simulink model "store"  (R2017b)
settings: Solver=VariableStepAuto  StartTime=0.0  StopTime=10.0  RelTol=1e-3
libraries: simulink x1
settings Model: Creator=Administrator  LastModifiedBy=Administrator

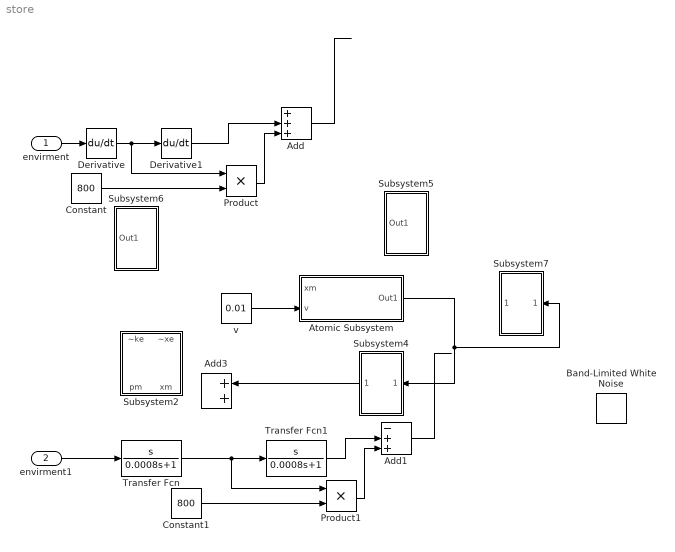
== system store ==
  envirment : Inport
  envirment1 : Inport  Port=2
  Add : Sum  Inputs=+++
  Add1 : Sum  Inputs=-++
  Add3 : Sum
  Atomic Subsystem : Subsystem  TreatAsAtomicUnit=on
  Band-Limited White Noise : simulink/Sources/Band-Limited White Noise  Cov=[0.000000005]  Ts=0.005  seed=[23341]
  Constant : Constant  Value=800
  Constant1 : Constant  Value=800
  Derivative : Derivative
  Derivative1 : Derivative
  Product : Product
  Product1 : Product
  Subsystem2 : Subsystem
  Subsystem4 : Subsystem
  Subsystem5 : Subsystem
  Subsystem6 : Subsystem
  Subsystem7 : Subsystem
  Transfer Fcn : TransferFcn  Numerator=[1 0]  Denominator=[0.0008 1]
  Transfer Fcn1 : TransferFcn  Numerator=[1 0]  Denominator=[0.0008 1]
  v : Constant  Value=0.01
  wires:
  v/1 -> Atomic Subsystem/2(v)
  Atomic Subsystem/1(Out1) -> Subsystem7/1(In1), Subsystem4/1(In1)
  Subsystem4/1(Out1) -> Add3/1
  envirment/1 -> Derivative/1
  ? -> Add/1
  Constant/1 -> Product/2
  Derivative/1 -> Product/1, Derivative1/1
  Add/1 -> ?
  Derivative1/1 -> Add/2
  Product/1 -> Add/3
  ? -> Add1/1
  envirment1/1 -> Transfer Fcn/1
  Transfer Fcn1/1 -> Add1/2
  Transfer Fcn/1 -> Transfer Fcn1/1, Product1/1
  Product1/1 -> Add1/3
  Add1/1 -> ?
  Constant1/1 -> Product1/2

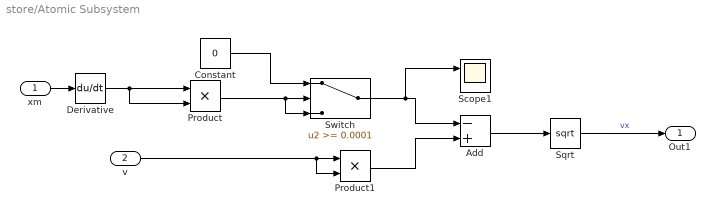
== system store/Atomic Subsystem ==
  xm : Inport
  v : Inport  Port=2
  Add : Sum  Inputs=-+
  Constant : Constant  Value=0
  Derivative : Derivative
  Product : Product
  Product1 : Product
  Scope1 : Scope  NumInputPorts=2
  Sqrt : Sqrt  SaturateOnIntegerOverflow=on
  Switch : Switch  Threshold=0.0001
  Out1 : Outport
  wires:
  xm/1 -> Derivative/1
  v/1 -> Product1/2, Product1/1
  Product1/1 -> Add/2
  Add/1 -> Sqrt/1
  Sqrt/1 -> Out1/1  "vx"
  Derivative/1 -> Product/2, Product/1
  Switch/1 -> Scope1/1, Add/1
  Constant/1 -> Switch/1
  Product/1 -> Switch/3, Switch/2

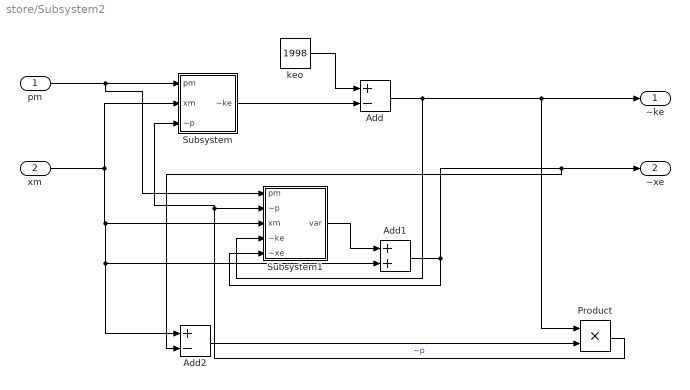
== system store/Subsystem2 ==
  pm : Inport
  xm : Inport  Port=2
  Add : Sum  Inputs=+-
  Add1 : Sum
  Add2 : Sum  Inputs=+-
  Product : Product
  Subsystem : Subsystem
  Subsystem1 : Subsystem
  keo : Constant  Value=1998
  ~ke : Outport
  ~xe : Outport  Port=2
  wires:
  pm/1 -> Subsystem1/1(pm), Subsystem/1(pm)
  xm/1 -> Subsystem/2(xm), Add1/2, Add2/1, Subsystem1/3(xm)
  Add/1 -> Subsystem1/4(~ke), Product/1, ~ke/1
  Subsystem/1(~ke) -> Add/2
  Subsystem1/1(var) -> Add1/1
  Add1/1 -> Subsystem1/5("~xe "), Add2/2, ~xe/1
  Add2/1 -> Product/2
  Product/1 -> Subsystem/3(~p), Subsystem1/2(~p)  "~p"
  keo/1 -> Add/1

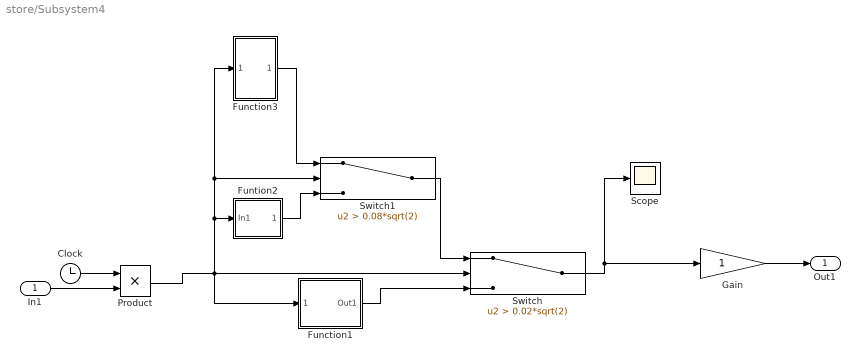
== system store/Subsystem4 ==
  In1 : Inport
  Clock : Clock
  Function1 : Subsystem
  Function3 : Subsystem
  Funtion2 : Subsystem
  Gain : Gain
  Product : Product
  Scope : Scope
  Switch : Switch  Criteria=u2 > Threshold  Threshold=0.02*sqrt(2)
  Switch1 : Switch  Criteria=u2 > Threshold  Threshold=0.08*sqrt(2)
  Out1 : Outport
  wires:
  Function3/1(Out1) -> Switch1/1
  Funtion2/1(Out1) -> Switch1/3
  Clock/1 -> Product/1
  Product/1 -> Function1/1(time in), Switch/2, Function3/1(In1), Switch1/2, Funtion2/1(In1)
  Switch1/1 -> Switch/1
  Switch/1 -> Gain/1, Scope/1
  Function1/1(Out1) -> Switch/3
  Gain/1 -> Out1/1
  In1/1 -> Product/2

== system store/Subsystem5 ==
  Clock : Clock
  Function1 : Subsystem
  Function3 : Subsystem
  Funtion2 : Subsystem
  Gain : Gain
  Gain1 : Gain  Gain=5/1000
  Scope : Scope
  Switch : Switch  Criteria=u2 > Threshold  Threshold=0.0282842712474619
  Switch1 : Switch  Criteria=u2 > Threshold  Threshold=0.1131370849898476
  Out1 : Outport
  wires:
  Gain/1 -> Out1/1
  Function1/1(Out1) -> Switch/3
  Switch/1 -> Scope/1, Gain/1
  Switch1/1 -> Switch/1
  Clock/1 -> Gain1/1
  Funtion2/1(Out1) -> Switch1/3
  Function3/1(Out1) -> Switch1/1
  Gain1/1 -> Funtion2/1(In1), Switch1/2, Function3/1(In1), Switch/2, Function1/1(time in)

== system store/Subsystem6 ==
  Clock : Clock
  Function1 : Subsystem
  Function3 : Subsystem
  Funtion2 : Subsystem
  Gain : Gain
  Gain1 : Gain  Gain=5/1000
  Scope : Scope
  Switch : Switch  Criteria=u2 > Threshold  Threshold=0.02*sqrt(2)
  Switch1 : Switch  Criteria=u2 > Threshold  Threshold=0.08*sqrt(2)
  Out1 : Outport
  wires:
  Gain/1 -> Out1/1
  Function1/1(Out1) -> Switch/3
  Switch/1 -> Scope/1, Gain/1
  Switch1/1 -> Switch/1
  Clock/1 -> Gain1/1
  Funtion2/1(Out1) -> Switch1/3
  Function3/1(Out1) -> Switch1/1
  Gain1/1 -> Funtion2/1(In1), Switch1/2, Function3/1(In1), Switch/2, Function1/1(time in)

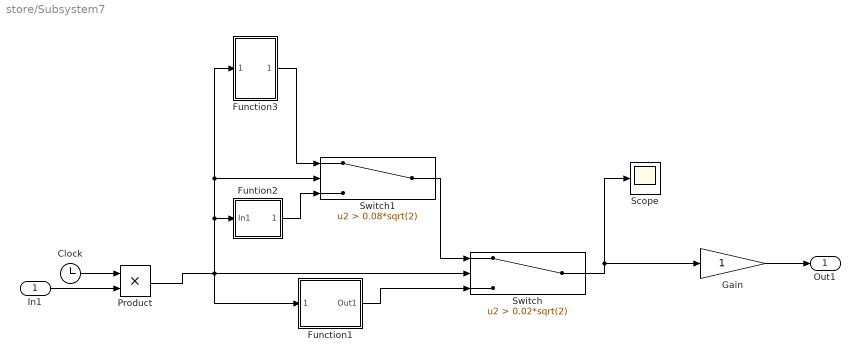
== system store/Subsystem7 ==
  In1 : Inport
  Clock : Clock
  Function1 : Subsystem
  Function3 : Subsystem
  Funtion2 : Subsystem
  Gain : Gain
  Product : Product
  Scope : Scope
  Switch : Switch  Criteria=u2 > Threshold  Threshold=0.02*sqrt(2)
  Switch1 : Switch  Criteria=u2 > Threshold  Threshold=0.08*sqrt(2)
  Out1 : Outport
  wires:
  In1/1 -> Product/2
  Gain/1 -> Out1/1
  Function1/1(Out1) -> Switch/3
  Switch/1 -> Scope/1, Gain/1
  Switch1/1 -> Switch/1
  Product/1 -> Funtion2/1(In1), Switch1/2, Function3/1(In1), Switch/2, Function1/1(time in)
  Clock/1 -> Product/1
  Funtion2/1(Out1) -> Switch1/3
  Function3/1(Out1) -> Switch1/1

== system store/Subsystem2/Subsystem ==
  pm : Inport
  xm : Inport  Port=2
  ~p : Inport  Port=3
  Add : Sum  Inputs=-+
  Integrator : Integrator
  Product : Product
  Product1 : Product
  Scope : Scope
  Subsystem1 : Subsystem
  ~ke : Outport
  wires:
  Subsystem1/2(γ2) -> Scope/1
  ~p/1 -> Add/2
  pm/1 -> Add/1
  xm/1 -> Product/1
  Add/1 -> Product/2
  Product/1 -> Integrator/1
  Integrator/1 -> Product1/2
  Product1/1 -> ~ke/1
  Subsystem1/1(γ1) -> Product1/1

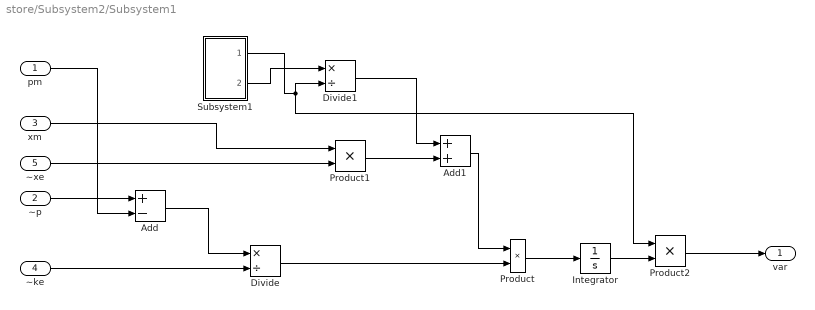
== system store/Subsystem2/Subsystem1 ==
  pm : Inport
  ~p : Inport  Port=2
  xm : Inport  Port=3
  ~ke : Inport  Port=4
  "~xe " : Inport  Port=5
  Add : Sum  Inputs=+-
  Add1 : Sum
  Divide : Product  Inputs=*/
  Divide1 : Product  Inputs=*/
  Integrator : Integrator
  Product : Product
  Product1 : Product
  Product2 : Product
  Subsystem1 : Subsystem
  var : Outport
  wires:
  pm/1 -> Add/2
  ~p/1 -> Add/1
  Add/1 -> Divide/1
  ~ke/1 -> Divide/2
  Divide/1 -> Product/2
  xm/1 -> Product1/1
  Divide1/1 -> Add1/1
  Product1/1 -> Add1/2
  Add1/1 -> Product/1
  Integrator/1 -> Product2/2
  Product2/1 -> var/1
  "~xe "/1 -> Product1/2
  Product/1 -> Integrator/1
  Subsystem1/2(gama2) -> Divide1/1
  Subsystem1/1(gama1) -> Product2/1, Divide1/2

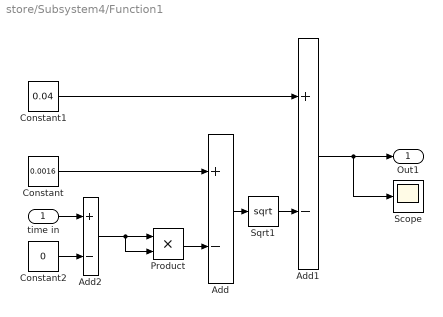
== system store/Subsystem4/Function1 ==
  time in : Inport
  Add : Sum  Inputs=+-
  Add1 : Sum  Inputs=+-
  Add2 : Sum  Inputs=+-
  Constant : Constant  Value=0.0016
  Constant1 : Constant  Value=0.04
  Constant2 : Constant  Value=0
  Product : Product
  Scope : Scope
  Sqrt1 : Sqrt  SaturateOnIntegerOverflow=on
  Out1 : Outport
  wires:
  Constant/1 -> Add/1
  time in/1 -> Add2/1
  Constant2/1 -> Add2/2
  Add2/1 -> Product/2, Product/1
  Product/1 -> Add/2
  Add/1 -> Sqrt1/1
  Sqrt1/1 -> Add1/2
  Constant1/1 -> Add1/1
  Add1/1 -> Out1/1, Scope/1

== system store/Subsystem4/Function3 ==
  In1 : Inport
  Add : Sum  Inputs=+-
  Add1 : Sum  Inputs=+-
  Add2 : Sum  Inputs=+-
  Product1 : Product
  Sqrt : Sqrt  SaturateOnIntegerOverflow=on
  pr2 : Constant  Value=0.0016
  pr3 : Constant  Value=0.1*sqrt(2)
  pr4 : Constant  Value=0.04
  Out1 : Outport
  wires:
  Add2/1 -> Out1/1
  pr3/1 -> Add1/2
  In1/1 -> Add1/1
  Add1/1 -> Product1/2, Product1/1
  Product1/1 -> Add/2
  pr2/1 -> Add/1
  Add/1 -> Sqrt/1
  pr4/1 -> Add2/1
  Sqrt/1 -> Add2/2

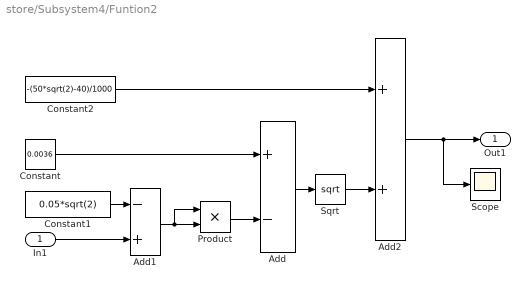
== system store/Subsystem4/Funtion2 ==
  In1 : Inport
  Add : Sum  Inputs=+-
  Add1 : Sum  Inputs=-+
  Add2 : Sum
  Constant : Constant  Value=0.0036
  Constant1 : Constant  Value=0.05*sqrt(2)
  Constant2 : Constant  Value=-(50*sqrt(2)-40)/1000
  Product : Product
  Scope : Scope
  Sqrt : Sqrt  SaturateOnIntegerOverflow=on
  Out1 : Outport
  wires:
  Constant/1 -> Add/1
  In1/1 -> Add1/2
  Add1/1 -> Product/1, Product/2
  Product/1 -> Add/2
  Constant1/1 -> Add1/1
  Add/1 -> Sqrt/1
  Sqrt/1 -> Add2/2
  Constant2/1 -> Add2/1
  Add2/1 -> Scope/1, Out1/1

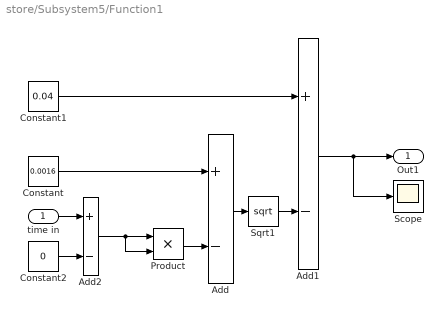
== system store/Subsystem5/Function1 ==
  time in : Inport
  Add : Sum  Inputs=+-
  Add1 : Sum  Inputs=+-
  Add2 : Sum  Inputs=+-
  Constant : Constant  Value=0.0016
  Constant1 : Constant  Value=0.04
  Constant2 : Constant  Value=0
  Product : Product
  Scope : Scope
  Sqrt1 : Sqrt  SaturateOnIntegerOverflow=on
  Out1 : Outport
  wires:
  Add1/1 -> Scope/1, Out1/1
  Constant1/1 -> Add1/1
  Sqrt1/1 -> Add1/2
  Add/1 -> Sqrt1/1
  Product/1 -> Add/2
  Add2/1 -> Product/1, Product/2
  Constant2/1 -> Add2/2
  time in/1 -> Add2/1
  Constant/1 -> Add/1

== system store/Subsystem5/Function3 ==
  In1 : Inport
  Add : Sum  Inputs=+-
  Add1 : Sum  Inputs=+-
  Add2 : Sum  Inputs=+-
  Product1 : Product
  Sqrt : Sqrt  SaturateOnIntegerOverflow=on
  pr2 : Constant  Value=0.0016
  pr3 : Constant  Value=0.14142135623731
  pr4 : Constant  Value=0.04
  Out1 : Outport
  wires:
  Sqrt/1 -> Add2/2
  pr4/1 -> Add2/1
  Add/1 -> Sqrt/1
  pr2/1 -> Add/1
  Product1/1 -> Add/2
  Add1/1 -> Product1/1, Product1/2
  In1/1 -> Add1/1
  pr3/1 -> Add1/2
  Add2/1 -> Out1/1

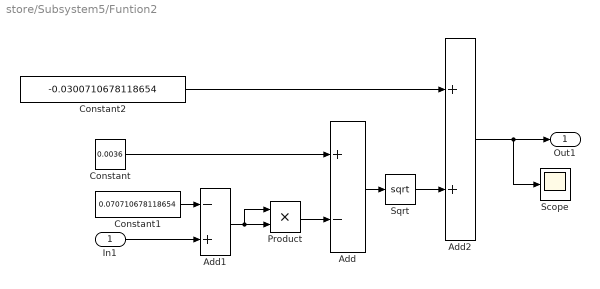
== system store/Subsystem5/Funtion2 ==
  In1 : Inport
  Add : Sum  Inputs=+-
  Add1 : Sum  Inputs=-+
  Add2 : Sum
  Constant : Constant  Value=0.0036
  Constant1 : Constant  Value=0.070710678118654
  Constant2 : Constant  Value=-0.0300710678118654
  Product : Product
  Scope : Scope
  Sqrt : Sqrt  SaturateOnIntegerOverflow=on
  Out1 : Outport
  wires:
  Add2/1 -> Out1/1, Scope/1
  Constant2/1 -> Add2/1
  Sqrt/1 -> Add2/2
  Add/1 -> Sqrt/1
  Constant1/1 -> Add1/1
  Product/1 -> Add/2
  Add1/1 -> Product/2, Product/1
  In1/1 -> Add1/2
  Constant/1 -> Add/1

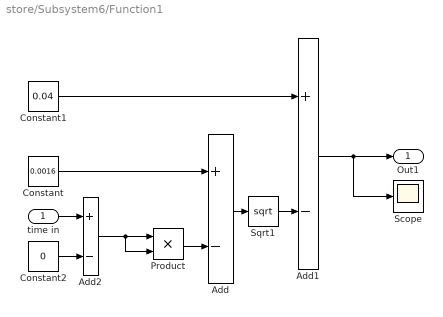
== system store/Subsystem6/Function1 ==
  time in : Inport
  Add : Sum  Inputs=+-
  Add1 : Sum  Inputs=+-
  Add2 : Sum  Inputs=+-
  Constant : Constant  Value=0.0016
  Constant1 : Constant  Value=0.04
  Constant2 : Constant  Value=0
  Product : Product
  Scope : Scope
  Sqrt1 : Sqrt  SaturateOnIntegerOverflow=on
  Out1 : Outport
  wires:
  Add1/1 -> Scope/1, Out1/1
  Constant1/1 -> Add1/1
  Sqrt1/1 -> Add1/2
  Add/1 -> Sqrt1/1
  Product/1 -> Add/2
  Add2/1 -> Product/1, Product/2
  Constant2/1 -> Add2/2
  time in/1 -> Add2/1
  Constant/1 -> Add/1

== system store/Subsystem6/Function3 ==
  In1 : Inport
  Add : Sum  Inputs=+-
  Add1 : Sum  Inputs=+-
  Add2 : Sum  Inputs=+-
  Product1 : Product
  Sqrt : Sqrt  SaturateOnIntegerOverflow=on
  pr2 : Constant  Value=0.0016
  pr3 : Constant  Value=0.1*sqrt(2)
  pr4 : Constant  Value=0.04
  Out1 : Outport
  wires:
  Sqrt/1 -> Add2/2
  pr4/1 -> Add2/1
  Add/1 -> Sqrt/1
  pr2/1 -> Add/1
  Product1/1 -> Add/2
  Add1/1 -> Product1/1, Product1/2
  In1/1 -> Add1/1
  pr3/1 -> Add1/2
  Add2/1 -> Out1/1

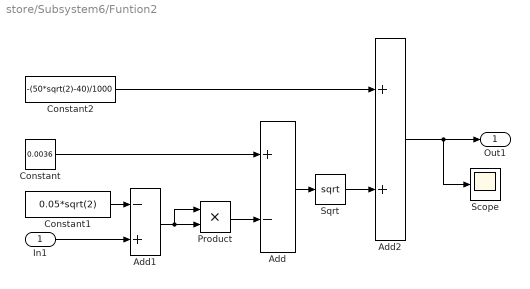
== system store/Subsystem6/Funtion2 ==
  In1 : Inport
  Add : Sum  Inputs=+-
  Add1 : Sum  Inputs=-+
  Add2 : Sum
  Constant : Constant  Value=0.0036
  Constant1 : Constant  Value=0.05*sqrt(2)
  Constant2 : Constant  Value=-(50*sqrt(2)-40)/1000
  Product : Product
  Scope : Scope
  Sqrt : Sqrt  SaturateOnIntegerOverflow=on
  Out1 : Outport
  wires:
  Add2/1 -> Out1/1, Scope/1
  Constant2/1 -> Add2/1
  Sqrt/1 -> Add2/2
  Add/1 -> Sqrt/1
  Constant1/1 -> Add1/1
  Product/1 -> Add/2
  Add1/1 -> Product/2, Product/1
  In1/1 -> Add1/2
  Constant/1 -> Add/1

== system store/Subsystem7/Function1 ==
  time in : Inport
  Add : Sum  Inputs=+-
  Add1 : Sum  Inputs=+-
  Add2 : Sum  Inputs=+-
  Constant : Constant  Value=0.0016
  Constant1 : Constant  Value=0.04
  Constant2 : Constant  Value=0
  Product : Product
  Scope : Scope
  Sqrt1 : Sqrt  SaturateOnIntegerOverflow=on
  Out1 : Outport
  wires:
  Add1/1 -> Scope/1, Out1/1
  Constant1/1 -> Add1/1
  Sqrt1/1 -> Add1/2
  Add/1 -> Sqrt1/1
  Product/1 -> Add/2
  Add2/1 -> Product/1, Product/2
  Constant2/1 -> Add2/2
  time in/1 -> Add2/1
  Constant/1 -> Add/1

== system store/Subsystem7/Function3 ==
  In1 : Inport
  Add : Sum  Inputs=+-
  Add1 : Sum  Inputs=+-
  Add2 : Sum  Inputs=+-
  Product1 : Product
  Sqrt : Sqrt  SaturateOnIntegerOverflow=on
  pr2 : Constant  Value=0.0016
  pr3 : Constant  Value=0.1*sqrt(2)
  pr4 : Constant  Value=0.04
  Out1 : Outport
  wires:
  Sqrt/1 -> Add2/2
  pr4/1 -> Add2/1
  Add/1 -> Sqrt/1
  pr2/1 -> Add/1
  Product1/1 -> Add/2
  Add1/1 -> Product1/1, Product1/2
  In1/1 -> Add1/1
  pr3/1 -> Add1/2
  Add2/1 -> Out1/1

== system store/Subsystem7/Funtion2 ==
  In1 : Inport
  Add : Sum  Inputs=+-
  Add1 : Sum  Inputs=-+
  Add2 : Sum
  Constant : Constant  Value=0.0036
  Constant1 : Constant  Value=0.05*sqrt(2)
  Constant2 : Constant  Value=-(50*sqrt(2)-40)/1000
  Product : Product
  Scope : Scope
  Sqrt : Sqrt  SaturateOnIntegerOverflow=on
  Out1 : Outport
  wires:
  Add2/1 -> Out1/1, Scope/1
  Constant2/1 -> Add2/1
  Sqrt/1 -> Add2/2
  Add/1 -> Sqrt/1
  Constant1/1 -> Add1/1
  Product/1 -> Add/2
  Add1/1 -> Product/2, Product/1
  In1/1 -> Add1/2
  Constant/1 -> Add/1

== system store/Subsystem2/Subsystem/Subsystem1 ==
  Demux : Demux  Outputs=2
  From Workspace : FromWorkspace  VariableName=simin  SampleTime=0
  Scope : Scope
  γ1 : Outport
  γ2 : Outport  Port=2
  wires:
  Demux/2 -> γ2/1
  Demux/1 -> γ1/1
  From Workspace/1 -> Scope/1, Demux/1

== system store/Subsystem2/Subsystem1/Subsystem1 ==
  Demux : Demux  Outputs=2
  From Workspace : FromWorkspace  VariableName=simin  SampleTime=0
  Scope : Scope
  gama1 : Outport
  gama2 : Outport  Port=2
  wires:
  Demux/2 -> gama2/1
  Demux/1 -> Scope/1, gama1/1
  From Workspace/1 -> Demux/1
